simulink model "gmskintdoc"  (Simulink 5.0)
settings: Solver=FixedStepDiscrete  StartTime=0.0  StopTime=2000.0  RelTol=1e-3
undefined symbols (not defined in the file or in its folder): rsgenpoly, slcm
libraries: commblkcod2 x2, commsink2 x2, commdigbbndcpm2 x2, commcnvintrlv2 x2, commchan2 x1, commrandsrc2 x1, dspsigops x1
settings Model: CovMetricSettings=d  Creator=mclune  LastModifiedBy=agaltman  SignalLoggingName=logsOut  BlockReductionOpt=off  BooleanDataType=off  ZeroCrossControl=UseLocalSettings  RTWMathFcnLibMatFile=iso_c_tmw.mat  RTWOptions="-aBlockComments=1 -aEnforceIntegerDowncast=1 -aExtMode=0 -aFoldNonRolledExpr=1 -aForceParamTrailComments=0 -aIgnoreCustomStorageClasses=1 -aInlineInvariantSignals=0 -aLocalBlockOutputs=1 -aLogVarNameModifier=\"rt_\" -aRTWVerbose=1 -aRollThreshold=5 -aShowEliminatedStatements=1"

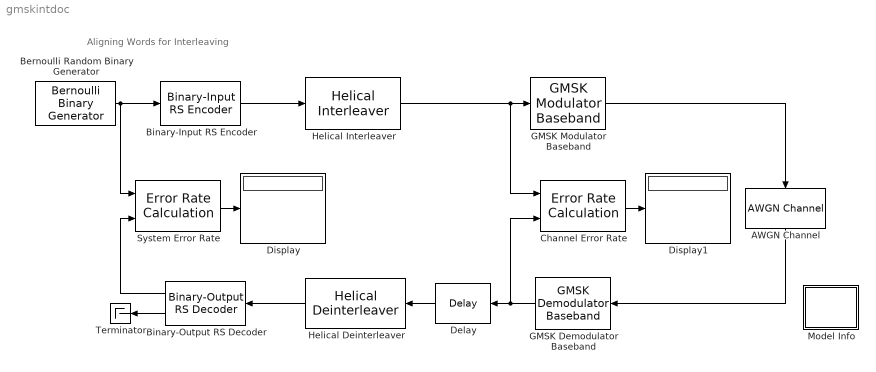
== system gmskintdoc ==
  note: Aligning Words for Interleaving
  AWGN Channel : commchan2/AWGN Channel  Orientation=down  seed=18233  noiseMode="Signal to noise ratio  (SNR)"  EsNodB=50  SNRdB=-6  Ps=1  Tsym=12  variance=1
  Bernoulli Random Binary Generator : commrandsrc2/Bernoulli Binary Generator  P=.5  seed=0  Ts=.1  frameBased=on  sampPerFrame=15  orient=off
  Binary-Input RS Encoder : commblkcod2/Binary-Input RS Encoder  n=7  k=5  specPrimPoly=off  primPoly=[1 0 1 1]  specGenPoly=off  genPoly=rsgenpoly(7,3)
  Binary-Output RS Decoder : commblkcod2/Binary-Output RS Decoder  Orientation=left  n=7  k=5  specPrimPoly=off  primPoly=[1 0 1 1]  specGenPoly=off  genPoly=rsgenpoly(7,3)  showNumErr=on
  Channel Error Rate : commsink2/Error Rate Calculation  N=16  st_delay=0  cp_mode=Entire frame  subframe=[]  PMode=Port  WsName=ErrorVec  RsMode2=off  stop=off  numErr=100  maxBits=1000
  Delay : dspsigops/Delay  Orientation=left  dly_unit=Samples  delay=5  ic_detail=off  dif_ic_for_ch=off  dif_ic_for_dly=off  ic=0  reset_popup=None
  Display : Display
  Display1 : Display
  GMSK Demodulator Baseband : commdigbbndcpm2/GMSK Demodulator Baseband  Orientation=left  OutputType=Bit  BT=.3  pulseLength=3  preHistory=1  phaseOffset=0  samplesPerSymbol=16  traceBack=16
  GMSK Modulator Baseband : commdigbbndcpm2/GMSK Modulator Baseband  inputType=Bit  BT=.3  pulseLength=3  preHistory=1  phaseOffset=0  samplesPerSymbol=16
  Helical Deinterleaver : commcnvintrlv2/Helical Deinterleaver  Orientation=left  C=7  N=3  s=1  ic=0
  Helical Interleaver : commcnvintrlv2/Helical Interleaver  C=7  N=3  s=1  ic=0
  Model Info : Subsystem  LoadFcn=slcm LoadBlock;  InitFcn=slcm('UpdateAllCMBlocksInThisModelInit')  mask(CMBlock){InitialSaveTempField=, InitialBlockCM=none, BlockCM=none, Frame=on, SaveTempField=, DisplayStringWithTags=Info, MaskDisplayString=Info, HorizontalTextAlignment=Center, LeftAlignmentValue=0.5, SourceBlockDiagram=gmskintdoc, TagMaxNumber=20, CMTag1=, CMTag2=, CMTag3=, CMTag4=, CMTag5=, CMTag6=, CMTag7=, CMTag8=, CMTag9=, CMTag10=, CMTag11=, CMTag12=, CMTag13=, CMTag14=, CMTag15=, CMTag16=, CMTag17=, CMTag18=, CMTag19=, CMTag20=}
      mask help: This block allows revision control information to be displayed within the model.
      settings: CopyFcn=slcm CopyBlock;  DeleteFcn=slcm Cancel;  PostSaveFcn=slcm('UpdateAllCMBlocksInThisModel')  NameChangeFcn=slcm Rename;  OpenFcn=commdemohelp;
      mask Display: text(str2num(LeftAlignmentValue), 0.5, MaskDisplayString, 'HorizontalAlignment', HorizontalTextAlignment)
  System Error Rate : commsink2/Error Rate Calculation  N=15*3  st_delay=0  cp_mode=Entire frame  subframe=[]  PMode=Port  WsName=ErrorVec  RsMode2=off  stop=off  numErr=100  maxBits=1000
  Terminator : Terminator
  wires:
  GMSK Modulator Baseband/1 -> AWGN Channel/1
  System Error Rate/1 -> Display/1
  AWGN Channel/1 -> GMSK Demodulator Baseband/1
  Bernoulli Random Binary Generator/1 -> System Error Rate/1, Binary-Input RS Encoder/1
  Delay/1 -> Helical Deinterleaver/1
  Helical Interleaver/1 -> Channel Error Rate/1, GMSK Modulator Baseband/1
  GMSK Demodulator Baseband/1 -> Channel Error Rate/2, Delay/1
  Binary-Input RS Encoder/1 -> Helical Interleaver/1
  Helical Deinterleaver/1 -> Binary-Output RS Decoder/1
  Binary-Output RS Decoder/1 -> System Error Rate/2
  Binary-Output RS Decoder/2 -> Terminator/1
  Channel Error Rate/1 -> Display1/1

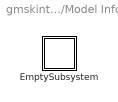
== system gmskintdoc/Model Info ==
  EmptySubsystem : Subsystem

== system gmskintdoc/Model Info/EmptySubsystem ==
